simulink model "maglev_bearing_platform"  (R2025a)
settings: Solver=ode4  StartTime=0.0  StopTime=5  FixedStep=1e-5  RelTol=1e-3  AbsTol=1e-3  EnableMultiTasking=on
InitFcn:
  | clear;
  | H = 0.035;
  | platform_radius = 0.1;
  | floater_hight = 0.03;
  | floater_radius = 0.01;
  | 
  | air_gap = 5.1e-4;
  | k_0 = 5.4414e-07;
  | 
  | Rz = @(th) [cos(th), -sin(th), 0; sin(th), cos(th), 0; 0, 0, 1];
  | Ry = @(th) [cos(th), 0, sin(th); 0, 1, 0; -sin(th), 0, cos(th)];
  | Rx = @(th) [1, 0, 0; 0, cos(th), -sin(th); 0, sin(th), cos(th)];
  | 
  | cross_matrix = @(a) [0, -a(3), a(2); a(3), 0, -a(1); -a(2), a(1), 0];
  | 
  | %% frame-platform to frame-mb0
  | R0 = Ry(deg2rad(-90)) * Rz(deg2rad(-90));
  | t0 = [(floater_hight * 0.5 + platform_radius); 0; -H];
  | 
  | T_mb0_2_platform = [R0, t0; 0, 0, 0, 1];
  | 
  | %% frame-platform to frame-mb1
  | R1 = Rz(deg2rad(-60)) * Ry(deg2rad(90)) * Rz(deg2rad(90));
  | t1 = [(floater_hight * 0.5 + platform_radius) * cos(pi/3*2); ...
  | (floater_hight * 0.5 + platform_radius) * sin(pi/3*2); -H];
  | 
  | T_mb1_2_platform = [R1, t1; 0, 0, 0, 1];
  | 
  | %% frame-platform to frame-mb2
  | 
  | R2 = Rz(deg2rad(60)) * Ry(deg2rad(90)) * Rz(deg2rad(90));
  | t2 = [(floater_hight * 0.5 + platform_radius) * cos(pi/3*4); ...
  | (floater_hight * 0.5 + platform_radius) * sin(pi/3*4); -H];
  | 
  | T_mb2_2_platform = [R2, t2; 0, 0, 0, 1];
  | 
  | %% mb0_fx, mb0_fy -> fx, fy, fz, tx, ty, tz
  | 
  | r0_fp = T_mb0_2_platform * [0 0 0 1]';
  | 
  | F0 = R0(:, 1:2);
  | 
  | T0 = cross_matrix(r0_fp) * R0;
  | T0 = T0(:, 1:2);
  | 
  | FT0 = [F0; T0];
  | 
  | %% mb1_fx, mb1_fy -> fx, fy, fz, tx, ty, tz
  | 
  | r1_fp = T_mb1_2_platform * [0 0 0 1]';
  | 
  | F1 = R1(:, 1:2);
  | 
  | T1 = cross_matrix(r1_fp) * R1;
  | T1 = T1(:, 1:2);
  | 
  | FT1 = [F1; T1];
  | 
  | %% mb2_fx, mb1_fy -> fx, fy, fz, tx, ty, tz
  | 
  | r2_fp = T_mb2_2_platform * [0 0 0 1]';
  | 
  | F2 = R2(:, 1:2);
  | 
  | T2 = cross_matrix(r2_fp) * R2;
  | T2 = T2(:, 1:2);
  | 
  | FT2 = [F2; T2];
  | 
  | % 局部坐标系到质心固连坐标系的转化
  | FT = [FT0 FT1 FT2];
undefined symbols (not defined in the file or in its folder): X, Y, Z
libraries: sm_lib x35, nesl_utility x17, simulink x1
(part 1 of 3)
settings Model: Creator=50263  LastModifiedBy=50263
settings SolverCC: AutoScaleAbsTol=off  AlgebraicLoopSolver=TrustRegion  AutoInsertRateTranBlk=on  MaxZcPerStep=1.0
settings DataIOCC: LimitDataPoints=on  MaxDataPoints=10000
settings OptimizationCC: ReuseModelBlockBuffer=off  LifeSpan=inf
settings DebuggingCC: UnconnectedInputMsg=warning  UnconnectedOutputMsg=warning  UnconnectedLineMsg=warning  AllowSymbolicDim=off  SubsystemReferenceDiagnosticForUnitTest=warning  SFUnexpectedBacktrackingDiag=warning  SFNoUnconditionalDefaultTransitionDiag=warning  SFExecutionAtInitializationDiag=none  ArithmeticOperatorsInVariantConditions=warning
settings ModelReferenceCC: EnableRefExpFcnMdlSchedulingChecks=on
settings SFSimCC: SimUseLocalCustomCode=off  CustomCodeUndefinedFunction=UseInterfaceOnly
settings RTWCC: RTWUseLocalCustomCode=off  GPUComputeCapability=3.5  DLArmComputeVersion=19.05
settings CodeAppCC: StateflowObjectComments=on
settings GRTTargetCC: TargetLangStandard=C89/C90 (ANSI)
settings ConfigComp: CovMetricSettings=dw  CovSaveCumulativeToWorkspaceVar=on  CovSaveSingleToWorkspaceVar=on  CovExternalEMLEnable=off  CovSFcnEnable=off
settings SimscapeCC: SimscapeLogType=all  SimscapeLogSimulationStatistics=on  SimscapeLogDataHistory=10000.0
settings ExplorerConfigSet: InternalSimMechanicsExplorerSettings=|
  | <ExplorerConfiguration>
  | 
  |   <canonicalview>default</canonicalview>
  | 
  |   <TilePanel>
  |     <TileInfo>
  |       <Tiles Columns="1" Count="1" Height="811" Rows="1" Width="1250">
  |         <Row Weight="1"/>
  |         <Column Weight="1"/>
  |         <Tile Height="1" Width="1" X="0" Y="0"/>
  |       </Tiles>
  |     </TileInfo>
  |     <SceneInfo>
  |       <SceneViewer>
  |         <IsThisViewStd>
  |           <IsStandardView>off</IsStandardView>
  |           <StandardViewName>Front</StandardViewName>
  |         </IsThisViewStd>
  |         <BGColor>
  |           <R>1</R>
  |           <G>1</G>
  |           <B>1</B>
  |           <A>1</A>
  |         </BGColor>
  |         <Camera>
  |           <DoPerspective>off</DoPerspective>
  |           <Position>
  |             <X>-0.50863418014720874</X>
  |             <Y>-0.75614907289451982</Y>
  |             <Z>0.036850771738493299</Z>
  |           </Position>
  |           <Center>
  |             <X>0.039683420290101482</X>
  |             <Y>0.12520259704718822</Y>
  |             <Z>0.03448179693193474</Z>
  |           </Center>
  |           <Up>
  |             <X>0.026099801835942574</X>
  |             <Y>-0.013550811679623347</Y>
  |             <Z>0.99956749439292392</Z>
  |           </Up>
  |           <XLim>0.095183756728403915</XLim>
  |           <YLim>0.095183756728403915</YLim>
  |           <ViewLimDist>0.01</ViewLimDist>
  |         </Camera>
  |       </SceneViewer>
  |     </SceneInfo>
  |   </TilePanel>
  | 
  |   <MechEditorPanel>
  |     <GfxPanelCameraMap/>
  |     <Cameras/>
  |     <VideoCreator>
  |       <IncludeTiles>All</IncludeTiles>
  |       <IncludeTime>on</IncludeTime>
  |       <IncludeWorldFrame>off</IncludeWorldFrame>
  |       <PlaybackSpeedRatio>1</PlaybackSpeedRatio>
  |       <FrameRate>30</FrameRate>
  |       <FrameSize>auto</FrameSize>
  |       <VideoFormat>UncompressedAVI</VideoFormat>
  |     </VideoCreator>
  |   </MechEditorPanel>
  | 
  |   <PlaybackSettings>
  |     <PlaybackSpeedFactor>0.25</PlaybackSpeedFactor>
  |   </PlaybackSettings>
  | 
  | </ExplorerConfiguration>

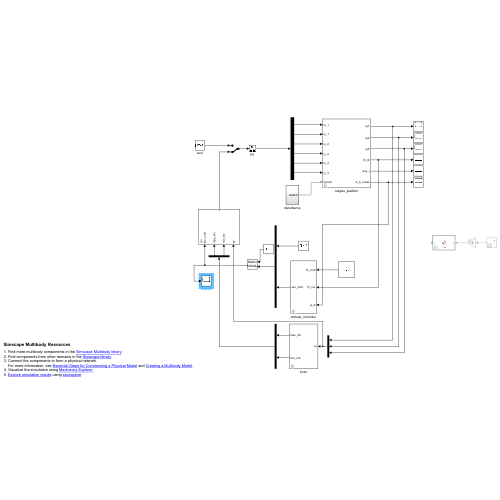
[thumbnail: Simulink's stored preview of the top-level diagram]
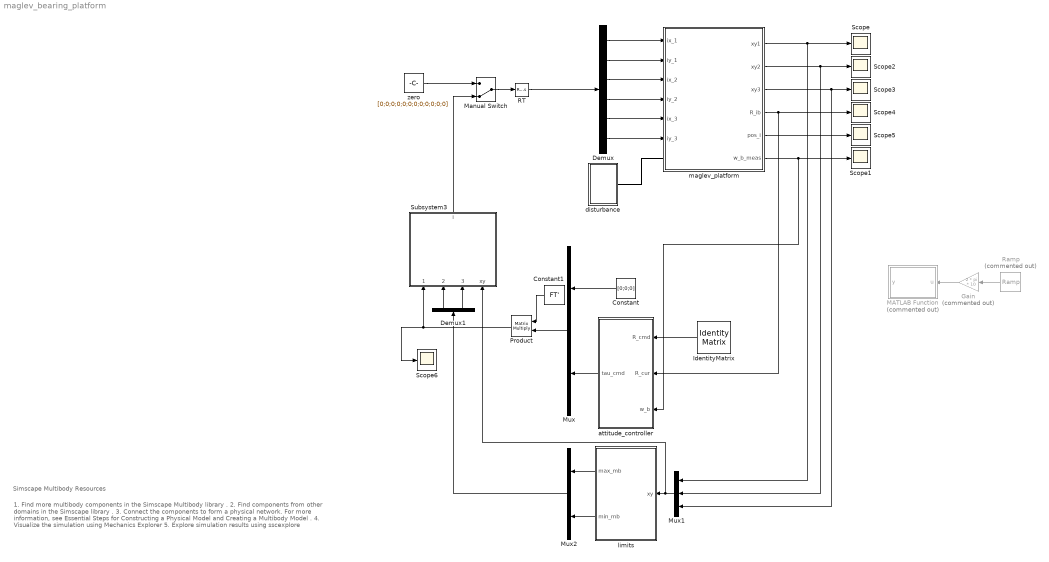
== system maglev_bearing_platform ==
  note: 1. Find more multibody components in the Simscape Multibody library .
      | 2. Find components from other domains in the Simscape library .
      | 3. Connect the components to form a physical network.
      | For more information, see Essential Steps for Constructing a Physical Model and Creating a Multibody Model .
      | 4. Visualize the simulation using Mechanics Explorer
      | 5. Explore simulation results using sscexplore
  note: Simscape Multibody Resources
  Constant : Constant  Value=[0;0;0]
  Constant1 : Constant  Value=FT'
  Demux : Demux  Outputs=6
  Demux1 : Demux  Outputs=2
  Gain : Gain  Commented=on  Gain=2 * pi * 10
  IdentityMatrix : IdentityMatrix  OutputDimensions=3
  MATLAB Function : MATLAB Function  Commented=on  TreatAsAtomicUnit=on
  Manual Switch : ManualSwitch  CurrentSetting=0
  Mux : Mux  Inputs=2
  Mux1 : Mux  Inputs=3
  Mux2 : Mux  Inputs=2
  Product : Product  Multiplication=Matrix(*)
  RT : RateTransition  OutPortSampleTime=1e-5
  Ramp : simulink/Sources/Ramp  Commented=on  slope=1  start=0  InitialOutput=0
  Scope{,1..6} (7 alike) : Scope
      Scope settings: ActiveDisplayYMinimum=-0.00061620865418658894  ActiveDisplayYMaximum=0.00053142107895254309
      Scope1 settings: ActiveDisplayYMinimum=-0.73841941905190533  ActiveDisplayYMaximum=0.40982335535694486  DataLoggingVariableName=ScopeData2
      Scope2 settings: ActiveDisplayYMinimum=-0.00062700637156377155  ActiveDisplayYMaximum=0.0006269831636385927  DataLoggingVariableName=ScopeData3
      Scope3 settings: ActiveDisplayYMinimum=-0.00062700637156377134  ActiveDisplayYMaximum=0.00062698316363859249  DataLoggingVariableName=ScopeData4
      Scope4 settings: ActiveDisplayYMinimum=-0.0036816071471794214  ActiveDisplayYMaximum=0.0027900662407171024
      Scope5 settings: ActiveDisplayYMinimum=-0.0075000003911005206  ActiveDisplayYMaximum=0.067500000043455868  DataLoggingVariableName=ScopeData5
      Scope6 settings: ActiveDisplayYMinimum=-26.030691483063197  ActiveDisplayYMaximum=26.603592648958866  DataLoggingVariableName=ScopeData6
  Subsystem3 : Subsystem  mask{k_0=k_0, air_gap=air_gap, i_max=6}
  attitude_controller : Subsystem  mask{Kp=5000, Kd=300}
  disturbance : Subsystem
  limits : Subsystem  mask{air_gap=air_gap, k_0=5.4414e-07, i_max=6}
  maglev_platform : Subsystem  mask{k_spring=5000, mech_gap=7e-4, R=0.025, H=H, platform_radius=platform_radius, floater_hight=floater_hight, floater_radius=floater_radius}
      mask prompts: k_spring "k_spring(N/m)"; mech_gap "mech_gap(m)"; R "R(Outer Diameter/m)"; H "H(Platform Lift Hight/m)"; platform_radius "R(m)"; floater_hight "Floater_H"; floater_radius "Floater_R"
      mask DialogControl Container3 Prompt: platform geometry
  zero : Constant  Value=[0;0;0;0;0;0;0;0;0;0;0;0]
  wires:
  maglev_platform/1(xy1) -> Scope/1, Mux1/1
  maglev_platform/2(xy2) -> Scope2/1, Mux1/2
  maglev_platform/3(xy3) -> Scope3/1, Mux1/3
  maglev_platform/4(R_ib) -> Scope4/1, attitude_controller/2(R_cur)
  maglev_platform/5(pos_i) -> Scope5/1
  Mux1/1 -> Subsystem3/4(xy), limits/1(xy)
  maglev_platform/6(w_b_meas) -> Scope1/1, attitude_controller/3(w_b)
  attitude_controller/1(tau_cmd) -> Mux/2
  Constant/1 -> Mux/1
  Mux/1 -> Product/2
  Constant1/1 -> Product/1
  Demux/1 -> maglev_platform/1(ix_1)
  Demux/2 -> maglev_platform/2(iy_1)
  Demux/3 -> maglev_platform/3(ix_2)
  Demux/4 -> maglev_platform/4(iy_2)
  Demux/5 -> maglev_platform/5(ix_3)
  Demux/6 -> maglev_platform/6(iy_3)
  Gain/1 -> MATLAB Function/1(u)
  Ramp/1 -> Gain/1
  IdentityMatrix/1 -> attitude_controller/1(R_cmd)
  Product/1 -> Scope6/1, Subsystem3/1(tau_cmd)
  limits/1(max_mb) -> Mux2/1
  limits/2(min_mb) -> Mux2/2
  Demux1/1 -> Subsystem3/2(max_lim)
  Demux1/2 -> Subsystem3/3(min_lim)
  Mux2/1 -> Demux1/1
  Subsystem3/1(i) -> Manual Switch/2
  RT/1 -> Demux/1
  Manual Switch/1 -> RT/1
  zero/1 -> Manual Switch/1
  connections:
  disturbance/RConn1 -- maglev_platform/LConn1

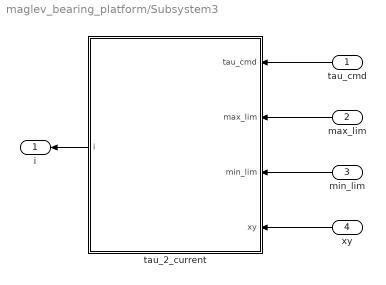
== system maglev_bearing_platform/Subsystem3 ==
  tau_cmd : Inport
  max_lim : Inport  Port=2
  min_lim : Inport  Port=3
  xy : Inport  Port=4
  tau_2_current : MATLAB Function  TreatAsAtomicUnit=on
  i : Outport
  wires:
  xy/1 -> tau_2_current/4(xy)
  min_lim/1 -> tau_2_current/3(min_lim)
  tau_2_current/1(i) -> i/1
  max_lim/1 -> tau_2_current/2(max_lim)
  tau_cmd/1 -> tau_2_current/1(tau_cmd)

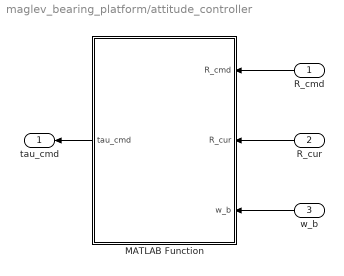
== system maglev_bearing_platform/attitude_controller ==
  R_cmd : Inport
  R_cur : Inport  Port=2
  w_b : Inport  Port=3
  MATLAB Function : MATLAB Function  TreatAsAtomicUnit=on  SystemSampleTime=1e-3
  tau_cmd : Outport
  wires:
  MATLAB Function/1(tau_cmd) -> tau_cmd/1
  w_b/1 -> MATLAB Function/3(w_b)
  R_cur/1 -> MATLAB Function/2(R_cur)
  R_cmd/1 -> MATLAB Function/1(R_cmd)

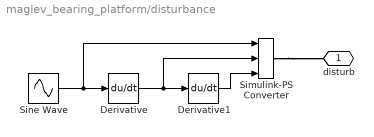
== system maglev_bearing_platform/disturbance ==
  Derivative : Derivative
  Derivative1 : Derivative
  Simulink-PS Converter : nesl_utility/Simulink-PS Converter  PhysicalDomain=network_engine_domain  SubClassName=ps_input  LeftPortType=input  RightPortType=output  PseudoPeriodic=off  Frequencies=[]  NoiseDistribution=none  NoiseParameters=[]  Unit=rad  AffineConversion=off  FilteringAndDerivatives=provide  SimscapeFilterOrder=1  InputFilterTimeConstant=0.001  UdotUserProvided=2
  Sine Wave : Sin  Amplitude=pi/180 * 0.2  Frequency=2*pi*10
  disturb : PMIOPort  Side=Right
  wires:
  Sine Wave/1 -> Simulink-PS Converter/1, Derivative/1
  Derivative/1 -> Derivative1/1, Simulink-PS Converter/2
  Derivative1/1 -> Simulink-PS Converter/3
  connections:
  Simulink-PS Converter/RConn1 -- disturb/RConn1

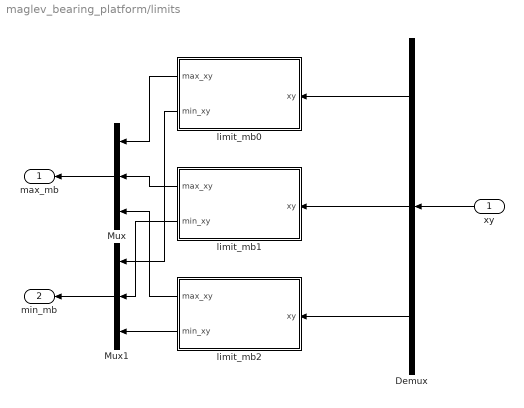
== system maglev_bearing_platform/limits ==
  xy : Inport
  Demux : Demux  Outputs=3
  Mux : Mux  Inputs=3
  Mux1 : Mux  Inputs=3
  limit_mb0 : MATLAB Function  TreatAsAtomicUnit=on
  limit_mb1 : MATLAB Function  TreatAsAtomicUnit=on
  limit_mb2 : MATLAB Function  TreatAsAtomicUnit=on
  max_mb : Outport
  min_mb : Outport  Port=2
  wires:
  Mux1/1 -> min_mb/1
  limit_mb0/2(min_xy) -> Mux1/1
  Demux/1 -> limit_mb0/1(xy)
  Mux/1 -> max_mb/1
  Demux/2 -> limit_mb1/1(xy)
  Demux/3 -> limit_mb2/1(xy)
  xy/1 -> Demux/1
  limit_mb0/1(max_xy) -> Mux/1
  limit_mb1/2(min_xy) -> Mux1/2
  limit_mb1/1(max_xy) -> Mux/2
  limit_mb2/2(min_xy) -> Mux1/3
  limit_mb2/1(max_xy) -> Mux/3
